simulink model "dmareference"  (R2020a)
settings: Solver=VariableStepAuto  StartTime=0.0  StopTime=inf  RelTol=1e-3
InitFcn:
  | dmareference_setup;
values from neighbouring files (symbols this model uses):
  f = 256e6    (= 256000000)    [dmareference_setup.m]
  Frames = 5    [dmareference_setup.m]
  PacketSize = 1024    [dmareference_setup.m]
libraries: simulink x6, hdlsllib x4, dspsrcs4 x1
settings Model: SimulationMode=accelerator  Creator=rgb11127  LastModifiedBy=david
settings DataIOCC: ReturnWorkspaceOutputs=off
settings DebuggingCC: ArithmeticOperatorsInVariantConditions=warning
settings SFSimCC: SimUseLocalCustomCode=off  CustomCodeUndefinedFunction=UseInterfaceOnly
settings RTWCC: RTWUseLocalCustomCode=off

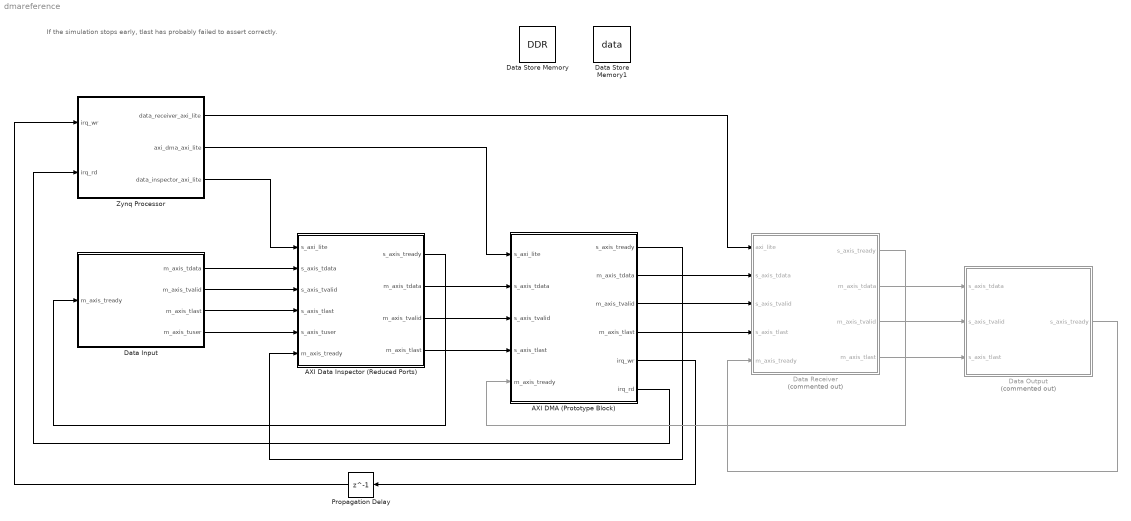
== system dmareference ==
  note: If the simulation stops early, tlast has probably failed to assert correctly.
  AXI DMA (Prototype Block) : Subsystem
  AXI Data Inspector (Reduced Ports) : Subsystem
  Data Input : Subsystem
  Data Output : Subsystem  Commented=on
  Data Receiver : Subsystem  Commented=on
  Data Store Memory : DataStoreMemory  DataStoreName=DDR  WriteAfterWriteMsg=warning  WriteAfterReadMsg=warning  ShowAdditionalParam=off  OutDataTypeStr=uint32  Dimensions=[hex2dec('FFFF')]
  Data Store Memory1 : DataStoreMemory  DataStoreName=data  WriteAfterWriteMsg=warning  WriteAfterReadMsg=warning  ShowAdditionalParam=off  OutDataTypeStr=uint32  Dimensions=[Frames, PacketSize]
  Propagation Delay : Delay  DelayLength=1
  Zynq Processor : Subsystem
  wires:
  AXI Data Inspector (Reduced Ports)/2(m_axis_tdata) -> AXI DMA (Prototype Block)/2(s_axis_tdata)
  AXI Data Inspector (Reduced Ports)/3(m_axis_tvalid) -> AXI DMA (Prototype Block)/3(s_axis_tvalid)
  AXI Data Inspector (Reduced Ports)/4(m_axis_tlast) -> AXI DMA (Prototype Block)/4(s_axis_tlast)
  AXI DMA (Prototype Block)/1(s_axis_tready) -> AXI Data Inspector (Reduced Ports)/6(m_axis_tready)
  AXI DMA (Prototype Block)/6(irq_rd) -> Zynq Processor/2(irq_rd)
  AXI DMA (Prototype Block)/5(irq_wr) -> Propagation Delay/1
  Zynq Processor/2(axi_dma_axi_lite) -> AXI DMA (Prototype Block)/1(s_axi_lite)
  Zynq Processor/3(data_inspector_axi_lite) -> AXI Data Inspector (Reduced Ports)/1(s_axi_lite)
  Data Input/1(m_axis_tdata) -> AXI Data Inspector (Reduced Ports)/2(s_axis_tdata)
  Data Input/2(m_axis_tvalid) -> AXI Data Inspector (Reduced Ports)/3(s_axis_tvalid)
  Data Input/3(m_axis_tlast) -> AXI Data Inspector (Reduced Ports)/4(s_axis_tlast)
  AXI Data Inspector (Reduced Ports)/1(s_axis_tready) -> Data Input/1(m_axis_tready)
  AXI DMA (Prototype Block)/2(m_axis_tdata) -> Data Receiver/2(s_axis_tdata)
  AXI DMA (Prototype Block)/3(m_axis_tvalid) -> Data Receiver/3(s_axis_tvalid)
  AXI DMA (Prototype Block)/4(m_axis_tlast) -> Data Receiver/4(s_axis_tlast)
  Zynq Processor/1(data_receiver_axi_lite) -> Data Receiver/1(axi_lite)
  Data Receiver/2(m_axis_tdata) -> Data Output/1(s_axis_tdata)
  Data Receiver/3(m_axis_tvalid) -> Data Output/2(s_axis_tvalid)
  Data Receiver/4(m_axis_tlast) -> Data Output/3(s_axis_tlast)
  Data Output/1(s_axis_tready) -> Data Receiver/5(m_axis_tready)
  Data Receiver/1(s_axis_tready) -> AXI DMA (Prototype Block)/5(m_axis_tready)
  Data Input/4(m_axis_tuser) -> AXI Data Inspector (Reduced Ports)/5(s_axis_tuser)
  Propagation Delay/1 -> Zynq Processor/1(irq_wr)

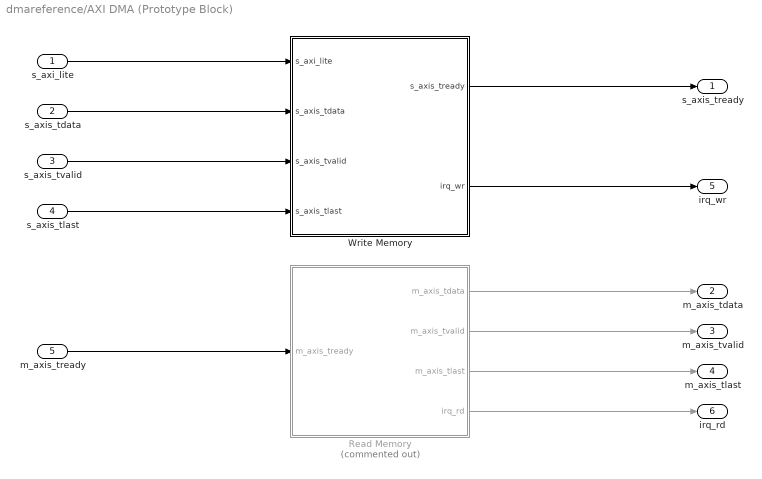
== system dmareference/AXI DMA (Prototype Block) ==
  s_axi_lite : Inport
  s_axis_tdata : Inport  Port=2
  s_axis_tvalid : Inport  Port=3
  s_axis_tlast : Inport  Port=4
  m_axis_tready : Inport  Port=5
  Read Memory : Subsystem  Commented=on
  Write Memory : Subsystem
  s_axis_tready : Outport  VectorParamsAs1DForOutWhenUnconnected=off
  m_axis_tdata : Outport  Port=2  VectorParamsAs1DForOutWhenUnconnected=off
  m_axis_tvalid : Outport  Port=3  VectorParamsAs1DForOutWhenUnconnected=off
  m_axis_tlast : Outport  Port=4  VectorParamsAs1DForOutWhenUnconnected=off
  irq_wr : Outport  Port=5  VectorParamsAs1DForOutWhenUnconnected=off
  irq_rd : Outport  Port=6  VectorParamsAs1DForOutWhenUnconnected=off
  wires:
  s_axis_tdata/1 -> Write Memory/2(s_axis_tdata)
  Read Memory/1(m_axis_tdata) -> m_axis_tdata/1
  s_axis_tvalid/1 -> Write Memory/3(s_axis_tvalid)
  s_axis_tlast/1 -> Write Memory/4(s_axis_tlast)
  Write Memory/1(s_axis_tready) -> s_axis_tready/1
  Read Memory/2(m_axis_tvalid) -> m_axis_tvalid/1
  Read Memory/3(m_axis_tlast) -> m_axis_tlast/1
  m_axis_tready/1 -> Read Memory/1(m_axis_tready)
  Write Memory/2(irq_wr) -> irq_wr/1
  Read Memory/4(irq_rd) -> irq_rd/1
  s_axi_lite/1 -> Write Memory/1(s_axi_lite)

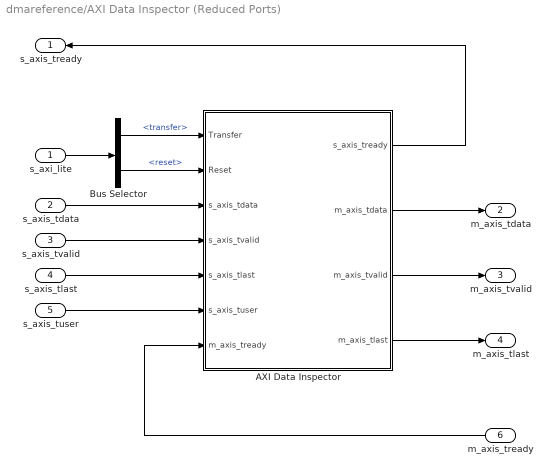
== system dmareference/AXI Data Inspector (Reduced Ports) ==
  s_axi_lite : Inport
  s_axis_tdata : Inport  Port=2
  s_axis_tvalid : Inport  Port=3
  s_axis_tlast : Inport  Port=4
  s_axis_tuser : Inport  Port=5
  m_axis_tready : Inport  Port=6
  AXI Data Inspector : Subsystem
  Bus Selector : BusSelector  OutputSignals=transfer,reset
  s_axis_tready : Outport  VectorParamsAs1DForOutWhenUnconnected=off
  m_axis_tdata : Outport  Port=2  VectorParamsAs1DForOutWhenUnconnected=off
  m_axis_tvalid : Outport  Port=3  VectorParamsAs1DForOutWhenUnconnected=off
  m_axis_tlast : Outport  Port=4  VectorParamsAs1DForOutWhenUnconnected=off
  wires:
  m_axis_tready/1 -> AXI Data Inspector/7(m_axis_tready)
  AXI Data Inspector/1(s_axis_tready) -> s_axis_tready/1
  AXI Data Inspector/2(m_axis_tdata) -> m_axis_tdata/1
  AXI Data Inspector/3(m_axis_tvalid) -> m_axis_tvalid/1
  AXI Data Inspector/4(m_axis_tlast) -> m_axis_tlast/1
  Bus Selector/1 -> AXI Data Inspector/1(Transfer)  "<transfer>"
  Bus Selector/2 -> AXI Data Inspector/2(Reset)  "<reset>"
  s_axi_lite/1 -> Bus Selector/1
  s_axis_tuser/1 -> AXI Data Inspector/6(s_axis_tuser)
  s_axis_tlast/1 -> AXI Data Inspector/5(s_axis_tlast)
  s_axis_tvalid/1 -> AXI Data Inspector/4(s_axis_tvalid)
  s_axis_tdata/1 -> AXI Data Inspector/3(s_axis_tdata)

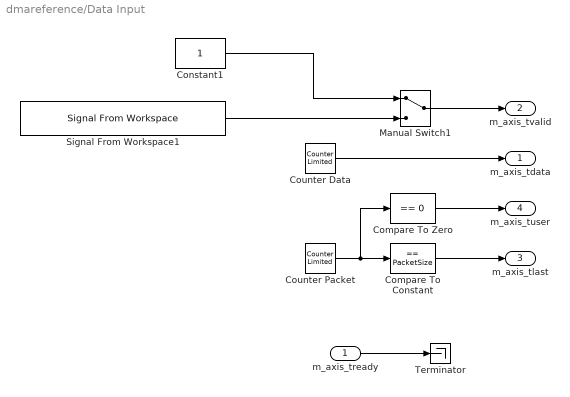
== system dmareference/Data Input ==
  m_axis_tready : Inport
  Compare To Constant : simulink/Logic and Bit Operations/Compare To Constant  relop===  const=PacketSize  OutDataTypeStr=boolean
  Compare To Zero : simulink/Logic and Bit Operations/Compare To Zero  relop===  OutDataTypeStr=boolean
  Constant1 : Constant  OutDataTypeStr=boolean  SampleTime=-1
  Counter Data : simulink/Sources/Counter Limited  uplimit=2^32-1  tsamp=1/f
  Counter Packet : simulink/Sources/Counter Limited  uplimit=PacketSize-1  tsamp=1/f
  Manual Switch1 : ManualSwitch
  Signal From Workspace1 : dspsrcs4/Signal From Workspace  X=[true(1,10000) false(1,2000) true(1, 10000)]  Ts=1/f  nsamps=1  OutputAfterFinalValue=Cyclic repetition  ignoreOrWarnInputAndFrameLengths=off  OutputFrames=off
  Terminator : Terminator
  m_axis_tdata : Outport  VectorParamsAs1DForOutWhenUnconnected=off
  m_axis_tvalid : Outport  Port=2  VectorParamsAs1DForOutWhenUnconnected=off
  m_axis_tlast : Outport  Port=3  VectorParamsAs1DForOutWhenUnconnected=off
  m_axis_tuser : Outport  Port=4  VectorParamsAs1DForOutWhenUnconnected=off
  wires:
  Constant1/1 -> Manual Switch1/1
  Signal From Workspace1/1 -> Manual Switch1/2
  Compare To Constant/1 -> m_axis_tlast/1
  Manual Switch1/1 -> m_axis_tvalid/1
  Counter Data/1 -> m_axis_tdata/1
  Counter Packet/1 -> Compare To Zero/1, Compare To Constant/1
  Compare To Zero/1 -> m_axis_tuser/1
  m_axis_tready/1 -> Terminator/1

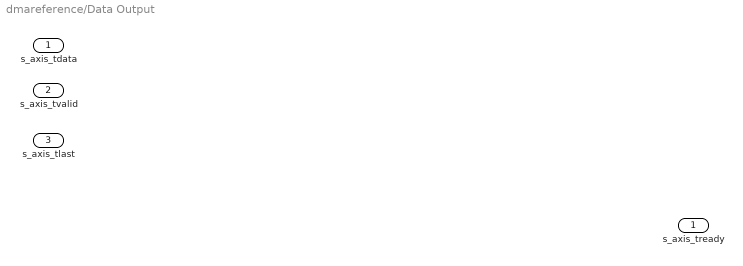
== system dmareference/Data Output ==
  s_axis_tdata : Inport
  s_axis_tvalid : Inport  Port=2
  s_axis_tlast : Inport  Port=3
  s_axis_tready : Outport  VectorParamsAs1DForOutWhenUnconnected=off

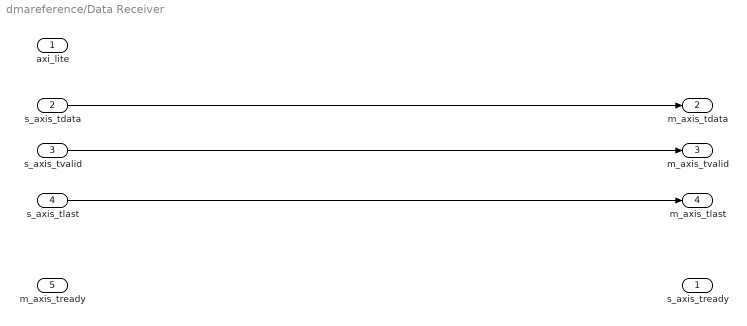
== system dmareference/Data Receiver ==
  axi_lite : Inport
  s_axis_tdata : Inport  Port=2
  s_axis_tvalid : Inport  Port=3
  s_axis_tlast : Inport  Port=4
  m_axis_tready : Inport  Port=5
  s_axis_tready : Outport  VectorParamsAs1DForOutWhenUnconnected=off
  m_axis_tdata : Outport  Port=2  VectorParamsAs1DForOutWhenUnconnected=off
  m_axis_tvalid : Outport  Port=3  VectorParamsAs1DForOutWhenUnconnected=off
  m_axis_tlast : Outport  Port=4  VectorParamsAs1DForOutWhenUnconnected=off
  wires:
  s_axis_tlast/1 -> m_axis_tlast/1
  s_axis_tvalid/1 -> m_axis_tvalid/1
  s_axis_tdata/1 -> m_axis_tdata/1

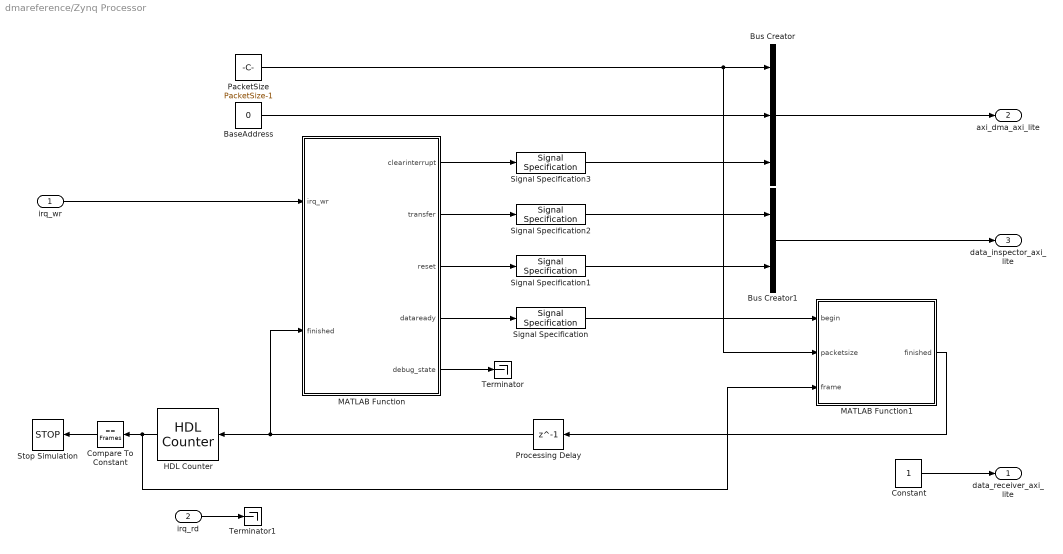
== system dmareference/Zynq Processor ==
  irq_wr : Inport
  irq_rd : Inport  Port=2
  BaseAddress : Constant  Value=0  OutDataTypeStr=uint32  SampleTime=-1
  Bus Creator : BusCreator  Inputs=3
  Bus Creator1 : BusCreator  Inputs=2
  Compare To Constant : simulink/Logic and Bit Operations/Compare To Constant  relop===  const=Frames  OutDataTypeStr=boolean
  Constant : Constant  SampleTime=-1
  HDL Counter : hdlsllib/Sources/HDL Counter  CountType=Free running  CountInit=0  CountStep=1  CountMax=25  CountFromType=Initial value  CountFrom=0  CountResetPort=off  CountLoadPort=off  CountEnbPort=on  CountDirPort=off  CountDataType=Unsigned  CountWordLen=8  CountFracLen=0  CountSampTime=1
  MATLAB Function : MATLAB Function  TreatAsAtomicUnit=on
  MATLAB Function1 : MATLAB Function  TreatAsAtomicUnit=on
  PacketSize : Constant  Value=PacketSize-1  OutDataTypeStr=uint32  SampleTime=-1
  Processing Delay : Delay  DelayLength=1
  Signal Specification{,1..3} (4 alike) : SignalSpecification  OutDataTypeStr=boolean
  Stop Simulation : Stop
  Terminator : Terminator
  Terminator1 : Terminator
  data_receiver_axi_lite : Outport  VectorParamsAs1DForOutWhenUnconnected=off
  axi_dma_axi_lite : Outport  Port=2  VectorParamsAs1DForOutWhenUnconnected=off
  data_inspector_axi_lite : Outport  Port=3  VectorParamsAs1DForOutWhenUnconnected=off
  wires:
  Bus Creator1/1 -> data_inspector_axi_lite/1
  Bus Creator/1 -> axi_dma_axi_lite/1
  MATLAB Function/2(transfer) -> Signal Specification2/1
  MATLAB Function/3(reset) -> Signal Specification1/1
  MATLAB Function/1(clearinterrupt) -> Signal Specification3/1
  irq_wr/1 -> MATLAB Function/1(irq_wr)
  PacketSize/1 -> MATLAB Function1/2(packetsize), Bus Creator/1
  BaseAddress/1 -> Bus Creator/2
  MATLAB Function/5(debug_state) -> Terminator/1
  irq_rd/1 -> Terminator1/1
  Constant/1 -> data_receiver_axi_lite/1
  MATLAB Function/4(dataready) -> Signal Specification/1
  MATLAB Function1/1(finished) -> Processing Delay/1
  Processing Delay/1 -> HDL Counter/1, MATLAB Function/2(finished)
  Signal Specification/1 -> MATLAB Function1/1(begin)
  Signal Specification1/1 -> Bus Creator1/2
  Signal Specification2/1 -> Bus Creator1/1
  Signal Specification3/1 -> Bus Creator/3
  HDL Counter/1 -> MATLAB Function1/3(frame), Compare To Constant/1
  Compare To Constant/1 -> Stop Simulation/1

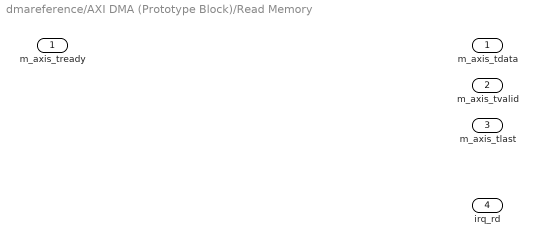
== system dmareference/AXI DMA (Prototype Block)/Read Memory ==
  m_axis_tready : Inport
  m_axis_tdata : Outport  VectorParamsAs1DForOutWhenUnconnected=off
  m_axis_tvalid : Outport  Port=2  VectorParamsAs1DForOutWhenUnconnected=off
  m_axis_tlast : Outport  Port=3  VectorParamsAs1DForOutWhenUnconnected=off
  irq_rd : Outport  Port=4  VectorParamsAs1DForOutWhenUnconnected=off

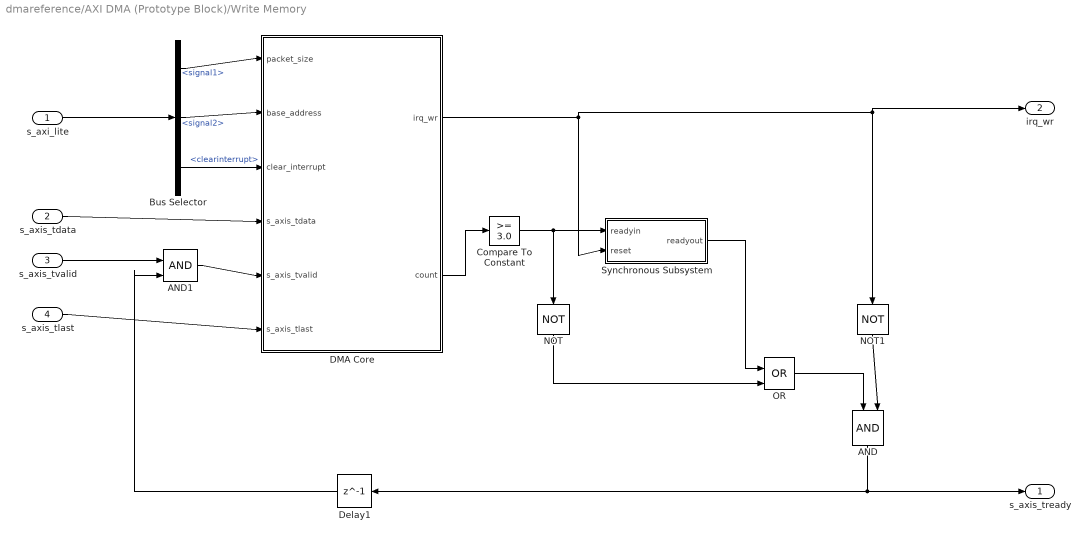
== system dmareference/AXI DMA (Prototype Block)/Write Memory ==
  s_axi_lite : Inport
  s_axis_tdata : Inport  Port=2
  s_axis_tvalid : Inport  Port=3
  s_axis_tlast : Inport  Port=4
  AND : Logic  IconShape=distinctive  AllPortsSameDT=off  OutDataTypeStr=boolean
  AND1 : Logic  IconShape=distinctive  AllPortsSameDT=off  OutDataTypeStr=boolean
  Bus Selector : BusSelector  OutputSignals=signal1,signal2,clearinterrupt
  Compare To Constant : simulink/Logic and Bit Operations/Compare To Constant  relop=>=  const=3.0  OutDataTypeStr=boolean
  DMA Core : Subsystem
  Delay1 : Delay  DelayLength=1
  NOT : Logic  Operator=NOT  IconShape=distinctive  AllPortsSameDT=off  OutDataTypeStr=boolean
  NOT1 : Logic  Operator=NOT  IconShape=distinctive  AllPortsSameDT=off  OutDataTypeStr=boolean
  OR : Logic  Operator=OR  IconShape=distinctive  AllPortsSameDT=off  OutDataTypeStr=boolean
  Synchronous Subsystem : Subsystem
  s_axis_tready : Outport  VectorParamsAs1DForOutWhenUnconnected=off
  irq_wr : Outport  Port=2  VectorParamsAs1DForOutWhenUnconnected=off
  wires:
  s_axis_tdata/1 -> DMA Core/4(s_axis_tdata)
  DMA Core/1(irq_wr) -> Synchronous Subsystem/2(reset), NOT1/1, irq_wr/1
  AND1/1 -> DMA Core/5(s_axis_tvalid)
  s_axis_tvalid/1 -> AND1/1
  s_axis_tlast/1 -> DMA Core/6(s_axis_tlast)
  DMA Core/2(count) -> Compare To Constant/1
  Compare To Constant/1 -> Synchronous Subsystem/1(readyin), NOT/1
  NOT/1 -> OR/2
  Synchronous Subsystem/1(readyout) -> OR/1
  Bus Selector/3 -> DMA Core/3(clear_interrupt)  "<clearinterrupt>"
  Bus Selector/2 -> DMA Core/2(base_address)  "<signal2>"
  Bus Selector/1 -> DMA Core/1(packet_size)  "<signal1>"
  s_axi_lite/1 -> Bus Selector/1
  Delay1/1 -> AND1/2
  AND/1 -> Delay1/1, s_axis_tready/1
  OR/1 -> AND/1
  NOT1/1 -> AND/2

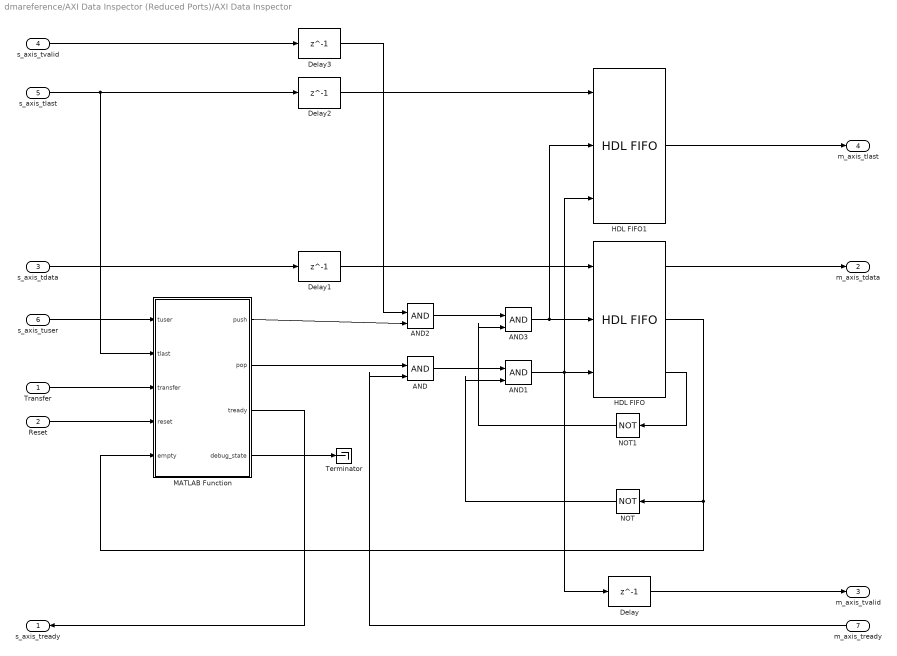
== system dmareference/AXI Data Inspector (Reduced Ports)/AXI Data Inspector ==
  Transfer : Inport
  Reset : Inport  Port=2
  s_axis_tdata : Inport  Port=3
  s_axis_tvalid : Inport  Port=4
  s_axis_tlast : Inport  Port=5
  s_axis_tuser : Inport  Port=6
  m_axis_tready : Inport  Port=7
  AND{,1..3} (4 alike) : Logic  IconShape=distinctive  AllPortsSameDT=off  OutDataTypeStr=boolean
  Delay{,1..3} (4 alike) : Delay  DelayLength=1  InitialCondition=0  UseCircularBuffer=on
  HDL FIFO : hdlsllib/HDL RAMs/HDL FIFO  fifo_size=MaxPacket  mode=Classic  ratio=1  push_msg=Error  pop_msg=Error  show_empty=on  show_full=on  show_num=off  LabelModeActiveChoice_Mode=Classic
      settings: SourceProductBaseCode=SL
  HDL FIFO1 : hdlsllib/HDL RAMs/HDL FIFO  fifo_size=MaxPacket  mode=Classic  ratio=1  push_msg=Error  pop_msg=Error  show_empty=off  show_full=off  show_num=off  LabelModeActiveChoice_Mode=Classic
      settings: SourceProductBaseCode=SL
  MATLAB Function : MATLAB Function  TreatAsAtomicUnit=on
  NOT : Logic  Operator=NOT  IconShape=distinctive  AllPortsSameDT=off  OutDataTypeStr=boolean
  NOT1 : Logic  Operator=NOT  IconShape=distinctive  AllPortsSameDT=off  OutDataTypeStr=boolean
  Terminator : Terminator
  s_axis_tready : Outport  VectorParamsAs1DForOutWhenUnconnected=off
  m_axis_tdata : Outport  Port=2  VectorParamsAs1DForOutWhenUnconnected=off
  m_axis_tvalid : Outport  Port=3  VectorParamsAs1DForOutWhenUnconnected=off
  m_axis_tlast : Outport  Port=4  VectorParamsAs1DForOutWhenUnconnected=off
  wires:
  m_axis_tready/1 -> AND/2
  Delay2/1 -> HDL FIFO1/1
  Transfer/1 -> MATLAB Function/3(transfer)
  AND/1 -> AND1/1
  s_axis_tlast/1 -> MATLAB Function/2(tlast), Delay2/1
  HDL FIFO/3 -> NOT1/1
  HDL FIFO/1 -> m_axis_tdata/1
  AND3/1 -> HDL FIFO1/2, HDL FIFO/2
  AND1/1 -> Delay/1, HDL FIFO1/3, HDL FIFO/3
  NOT1/1 -> AND3/2
  HDL FIFO/2 -> MATLAB Function/5(empty), NOT/1
  MATLAB Function/2(pop) -> AND/1
  NOT/1 -> AND1/2
  AND2/1 -> AND3/1
  s_axis_tdata/1 -> Delay1/1
  s_axis_tvalid/1 -> Delay3/1
  s_axis_tuser/1 -> MATLAB Function/1(tuser)
  Delay/1 -> m_axis_tvalid/1
  MATLAB Function/4(debug_state) -> Terminator/1
  Delay3/1 -> AND2/1
  Reset/1 -> MATLAB Function/4(reset)
  MATLAB Function/3(tready) -> s_axis_tready/1
  HDL FIFO1/1 -> m_axis_tlast/1
  Delay1/1 -> HDL FIFO/1
  MATLAB Function/1(push) -> AND2/2

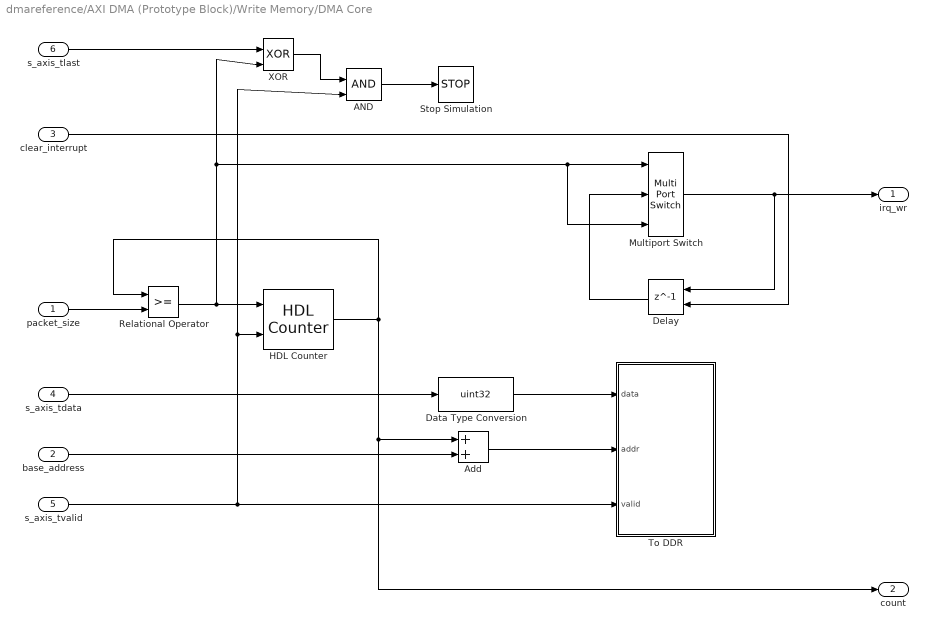
== system dmareference/AXI DMA (Prototype Block)/Write Memory/DMA Core ==
  packet_size : Inport
  base_address : Inport  Port=2
  clear_interrupt : Inport  Port=3
  s_axis_tdata : Inport  Port=4
  s_axis_tvalid : Inport  Port=5
  s_axis_tlast : Inport  Port=6
  AND : Logic  IconShape=distinctive  AllPortsSameDT=off  OutDataTypeStr=boolean
  Add : Sum  OutDataTypeStr=uint32
  Data Type Conversion : DataTypeConversion  OutDataTypeStr=uint32  ConvertRealWorld=Stored Integer (SI)
  Delay : Delay  DelayLength=1  ExternalReset=Level
      settings: InputPortMap=u0,r5
  HDL Counter : hdlsllib/Sources/HDL Counter  CountType=Free running  CountInit=0  CountStep=1  CountMax=25  CountFromType=Initial value  CountFrom=0  CountResetPort=on  CountLoadPort=off  CountEnbPort=on  CountDirPort=off  CountDataType=Unsigned  CountWordLen=32  CountFracLen=0  CountSampTime=1
  Multiport Switch : MultiPortSwitch  DataPortOrder=Zero-based contiguous  Inputs=2  zeroidx=on
  Relational Operator : RelationalOperator  OutDataTypeStr=boolean  RndMeth=Simplest
  Stop Simulation : Stop
  To DDR : MATLAB Function  TreatAsAtomicUnit=on
  XOR : Logic  Operator=XOR  IconShape=distinctive  AllPortsSameDT=off  OutDataTypeStr=boolean
  irq_wr : Outport  VectorParamsAs1DForOutWhenUnconnected=off
  count : Outport  Port=2  VectorParamsAs1DForOutWhenUnconnected=off
  wires:
  Add/1 -> To DDR/2(addr)
  Relational Operator/1 -> XOR/2, Multiport Switch/3, Multiport Switch/1, HDL Counter/1
  HDL Counter/1 -> count/1, Add/1, Relational Operator/1
  packet_size/1 -> Relational Operator/2
  s_axis_tvalid/1 -> AND/2, HDL Counter/2, To DDR/3(valid)
  Data Type Conversion/1 -> To DDR/1(data)
  base_address/1 -> Add/2
  s_axis_tdata/1 -> Data Type Conversion/1
  Multiport Switch/1 -> Delay/1, irq_wr/1
  Delay/1 -> Multiport Switch/2
  clear_interrupt/1 -> Delay/2
  s_axis_tlast/1 -> XOR/1
  XOR/1 -> AND/1
  AND/1 -> Stop Simulation/1

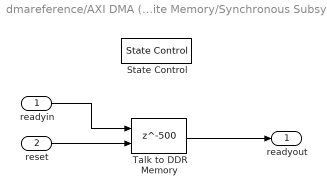
== system dmareference/AXI DMA (Prototype Block)/Write Memory/Synchronous Subsystem ==
  readyin : Inport
  reset : Inport  Port=2
  State Control : StateControl  StateControl=Synchronous
  Talk to DDR Memory : Delay  DelayLength=500  ExternalReset=Level
      settings: InputPortMap=u0,r5
  readyout : Outport  VectorParamsAs1DForOutWhenUnconnected=off
  wires:
  readyin/1 -> Talk to DDR Memory/1
  Talk to DDR Memory/1 -> readyout/1
  reset/1 -> Talk to DDR Memory/2

== matlab function dmareference/AXI Data Inspector (Reduced Ports)/AXI Data Inspector/MATLAB Function ==
  data: tuser input; push output; tlast input; transfer input; pop output; tready output; reset input; debug_state output; empty input
function [push, pop, tready, debug_state] = fcn(tuser, tlast, transfer, reset, empty)

IDLE = fi(0, 0, 2, 0);
TRANSFER = fi(1, 0, 2, 0);
PUSH = fi(2, 0, 2, 0);
RESET = fi(3, 0, 2, 0);

persistent state;

if isempty(state)
    state = IDLE;
end

switch state
    case IDLE
        push = false;
        pop = false;
        tready = true;
        debug_state = state;
        
        if tuser && transfer
            state = TRANSFER;
        else
            state = IDLE;
        end
        
    case TRANSFER
        push = true;
        pop = true;
        tready = true;
        debug_state = state;
        
        if tlast
            state = PUSH;
        else
            state = TRANSFER;
        end
        
    case PUSH
        push = true;
        pop = true;
        tready = false;
        debug_state = state;
        
        state = RESET;
        
    case RESET
        push = false;
        pop = true;
        tready = false;
        debug_state = state;
        
        if reset && empty
            state = IDLE;
        else
            state = RESET;
        end
        
        
    otherwise
        push = false;
        pop = false;
        tready = false;
        debug_state = state;
        
        state = IDLE;        
end

== matlab function dmareference/AXI DMA (Prototype Block)/Write Memory/DMA Core/To DDR ==
  data: data input; addr input; valid input; DDR data_store_memory
function fcn(data, addr, valid)

global DDR;

if valid
    DDR(addr+1) = data;
end

== matlab function dmareference/Zynq Processor/MATLAB Function ==
  data: irq_wr input; clearinterrupt output; transfer output; reset output; dataready output; finished input; debug_state output
function [clearinterrupt, transfer, reset, dataready, debug_state] = fcn(irq_wr, finished)

IDLE = fi(0, 0, 3, 0);
DMA = fi(1, 0, 3, 0);
INSP = fi(2, 0, 3, 0);
WAIT = fi(3, 0, 3, 0);
POST = fi(4, 0, 3, 0);
POST_2 = fi(7, 0, 3, 0);

persistent state;

if isempty(state)
    state = IDLE;
end

switch state
    case IDLE
        clearinterrupt = true;
        transfer = false;
        reset = true;
        dataready = false;
        debug_state = state;
        
        state = DMA;
        
    case DMA
        clearinterrupt = false;
        transfer = false;
        reset = true;
        dataready = false;
        debug_state = state;
        
        state = INSP;
        
    case INSP
        clearinterrupt = false;
        transfer = true;
        reset = false;
        dataready = false;
        debug_state = state;
        
        state = WAIT;
        
    case WAIT
        clearinterrupt = false;
        transfer = true;
        reset = false;
        dataready = false;
        debug_state = state;
        
        if irq_wr
            state = POST;
        else
            state = WAIT;
        end
        
    case POST
        clearinterrupt = false;
        transfer = false;
        reset = false;
        dataready = true;
        debug_state = state;
        
        state = POST_2;
        
    case POST_2
        clearinterrupt = false;
        transfer = false;
        reset = false;
        dataready = false;
        debug_state = state;
        
        if finished
            state = IDLE;
        else
            state = POST_2;
        end
        
    otherwise
        clearinterrupt = true;
        transfer = false;
        reset = true;
        dataready = false;
        debug_state = state;
        
        state = IDLE;
        
end

== matlab function dmareference/Zynq Processor/MATLAB Function1 ==
  data: begin input; finished output; packetsize input; DDR data_store_memory; frame input; data data_store_memory
function finished = fcn(begin, packetsize, frame)

coder.extrinsic('assignin');

global DDR;
global data;

if begin
    for i=1:packetsize+1
        data(frame+1, i) = DDR(i);
    end
    assignin('base', 'data', data);
    assignin('base', 'ddr', DDR);
    finished = true;
else
    finished = false;
end


end
